simulink model "Posture_Regulation_Singularity_ROS"  (R2022b)
settings: Solver=FixedStepAuto  StartTime=0.0  StopTime=inf  FixedStep=0.02  MaxStep=0.1  RelTol=1e-3
undefined symbols (not defined in the file): theta_f, unicycle, X, x_f, Y, y_f
libraries: robotlib x3, simulink_extras x2
settings Model: Creator=Musta  LastModifiedBy=Musta
settings OptimizationCC: EnhancedBackFolding=on  PassReuseOutputArgsAs=Individual arguments  ZeroExternalMemoryAtStartup=off  ZeroInternalMemoryAtStartup=off  MaxStackSize=64  OptimizeBlockOrder=speed  DifferentSizesBufferReuse=on  OptimizationCustomize=off  EfficientTunableParamExpr=on
settings DebuggingCC: ParameterTunabilityLossMsg=error
settings HardwareCC: ProdBitPerPointer=32  ProdBitPerSizeT=32  ProdBitPerPtrDiffT=32  ProdLargestAtomicFloat=None  ProdIntDivRoundTo=Undefined  ProdEndianess=Unspecified  ProdWordSize=32  ProdHWDeviceType=Generic->Unspecified (assume 32-bit Generic)
settings SFSimCC: MATLABDynamicMemAlloc=off
settings RTWCC: Description=Embedded Coder  SystemTargetFile=ert.tlc  HardwareBoard=Robot Operating System (ROS)  TLCOptions="-aInlineSetEventsForThisBaseRateFcn=TLC_FALSE -aSuppressMultiTaskScheduler=TLC_FALSE  -aRateBasedStepFcn=0"  TemplateMakefile=ert_default_tmf  Toolchain=Catkin  TargetLang=C++
settings CodeAppCC: ForceParamTrailComments=on  IgnoreCustomStorageClasses=off  OperatorAnnotations=on  SimulinkDataObjDesc=on  SFDataObjDesc=on  InsertBlockDesc=on

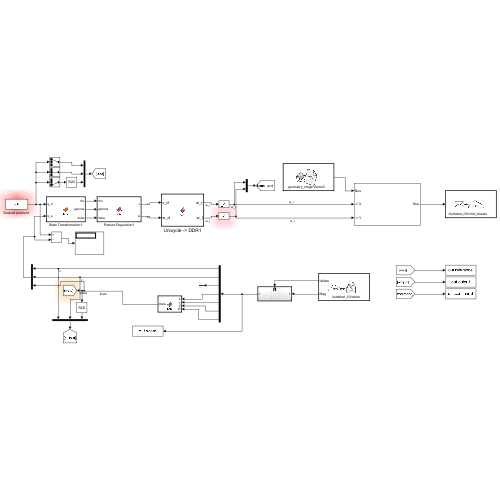
[thumbnail: Simulink's stored preview of the top-level diagram]
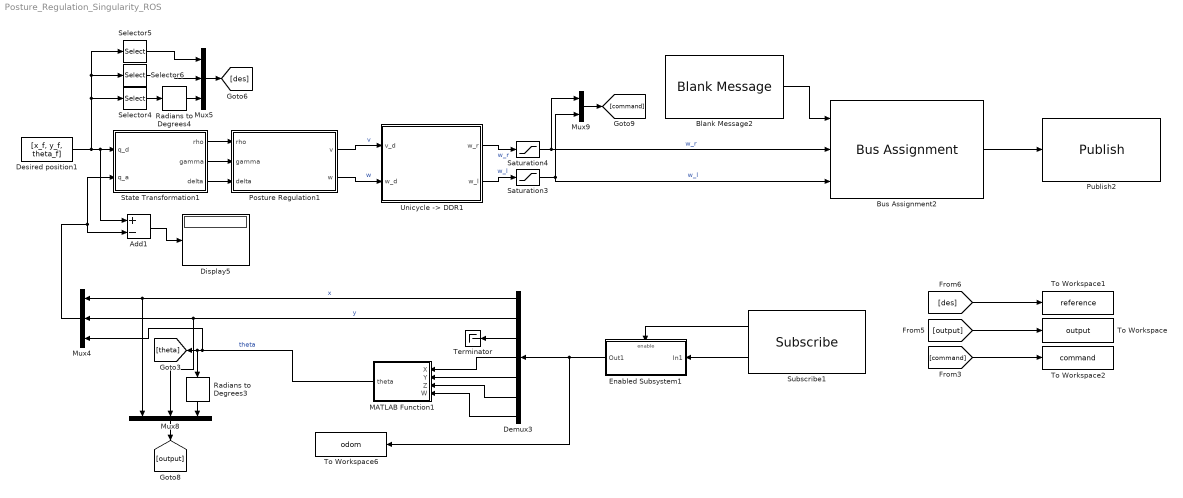
== system Posture_Regulation_Singularity_ROS ==
  Add1 : Sum  Inputs=+-
  Blank Message2 : robotlib/Blank Message  messageClass=Message  entityType=geometry_msgs/Vector3  messageType=geometry_msgs/Vector3  SampleTime=0.02  legacyBusStruct=off
      settings: LibrarySourceBlock=roslib/ROS/Blank Message
  Bus Assignment2 : BusAssignment  AssignedSignals=X,Y
  Demux3 : Demux  Outputs=7
  Desired position1 : Constant  Value=[x_f, y_f, theta_f]
  Display5 : Display
  Enabled Subsystem1 : Subsystem  TreatAsAtomicUnit=on
  MATLAB Function1 : MATLAB Function  TreatAsAtomicUnit=on
  Mux4 : Mux  Inputs=3
  Mux5 : Mux  Inputs=3
  Mux8 : Mux  Inputs=3
  Mux9 : Mux  Inputs=2
  Posture Regulation1 : MATLAB Function  TreatAsAtomicUnit=on
  Publish2 : robotlib/Publish  topicSource=Select from ROS network  topic=/turtlebot_03/cmd_wheels  messageType=geometry_msgs/Vector3  legacyBusStruct=off  messageQueueLength=1
      settings: LibrarySourceBlock=roslib/ROS/Publish
  Radians to Degrees3 : simulink_extras/Transformations/Radians to Degrees
  Radians to Degrees4 : simulink_extras/Transformations/Radians to Degrees
  Saturation3 : Saturate  UpperLimit=unicycle.omegaWheelMax  LowerLimit=unicycle.omegaWheelMin
  Saturation4 : Saturate  UpperLimit=13  LowerLimit=-13
  Selector4 : Selector  InputPortWidth=3  IndexOptions=Index vector (dialog)  Indices=3  OutputSizes=1
  Selector5 : Selector  InputPortWidth=3  IndexOptions=Index vector (dialog)  Indices=1  OutputSizes=1
  Selector6 : Selector  InputPortWidth=3  IndexOptions=Index vector (dialog)  Indices=2  OutputSizes=1
  State Transformation1 : MATLAB Function  TreatAsAtomicUnit=on
  Subscribe1 : robotlib/Subscribe  topicSource=Select from ROS network  topic=/turtlebot_03/odom  messageType=nav_msgs/Odometry  SampleTime=0.02  legacyBusStruct=off  messageQueueLength=1
      settings: LibrarySourceBlock=roslib/ROS/Subscribe
  Terminator : Terminator
  To Workspace : ToWorkspace  VariableName=output  SaveFormat=Structure With Time  SampleTime=-1
  To Workspace1 : ToWorkspace  VariableName=reference  SaveFormat=Structure With Time  SampleTime=-1
  To Workspace2 : ToWorkspace  VariableName=command  SaveFormat=Structure With Time  SampleTime=-1
  To Workspace6 : ToWorkspace  VariableName=odom  SaveFormat=Structure With Time  SampleTime=-1
  "Unicycle -> DDR1" : MATLAB Function  TreatAsAtomicUnit=on
  wires:
  [output] -> To Workspace/1
  [command] -> To Workspace2/1
  [des] -> To Workspace1/1
  Subscribe1/2 -> Enabled Subsystem1/1(In1)
  Enabled Subsystem1/1(Out1) -> Demux3/1, To Workspace6/1
  Subscribe1/1 -> Enabled Subsystem1/Enable
  MATLAB Function1/1(theta) -> Mux4/3, Radians to Degrees3/1, [theta]  "theta"
  Demux3/3 -> Terminator/1
  State Transformation1/1(rho) -> Posture Regulation1/1(rho)
  Demux3/1 -> Mux4/1, Mux8/1  "x"
  Selector5/1 -> Mux5/1
  Selector6/1 -> Mux5/2
  Radians to Degrees4/1 -> Mux5/3
  Mux5/1 -> [des]
  Bus Assignment2/1 -> Publish2/1
  Radians to Degrees3/1 -> Mux8/3
  Add1/1 -> Display5/1
  Demux3/2 -> Mux8/2, Mux4/2  "y"
  Posture Regulation1/1(v) -> "Unicycle -> DDR1"/1(v_d)  "v"
  Desired position1/1 -> Selector5/1, Selector6/1, Selector4/1, Add1/1, State Transformation1/1(q_d)
  Selector4/1 -> Radians to Degrees4/1
  State Transformation1/2(gamma) -> Posture Regulation1/2(gamma)
  Saturation4/1 -> Mux9/1, Bus Assignment2/2  "w_r"
  Mux4/1 -> State Transformation1/2(q_a), Add1/2
  Saturation3/1 -> Bus Assignment2/3, Mux9/2  "w_l"
  "Unicycle -> DDR1"/1(w_r) -> Saturation4/1  "w_r"
  Blank Message2/1 -> Bus Assignment2/1
  State Transformation1/3(delta) -> Posture Regulation1/3(delta)
  Posture Regulation1/2(w) -> "Unicycle -> DDR1"/2(w_d)  "w"
  Mux8/1 -> [output]
  "Unicycle -> DDR1"/2(w_l) -> Saturation3/1  "w_l"
  Mux9/1 -> [command]
  Demux3/5 -> MATLAB Function1/2(Y)
  Demux3/6 -> MATLAB Function1/3(Z)
  Demux3/4 -> MATLAB Function1/1(X)
  Demux3/7 -> MATLAB Function1/4(W)

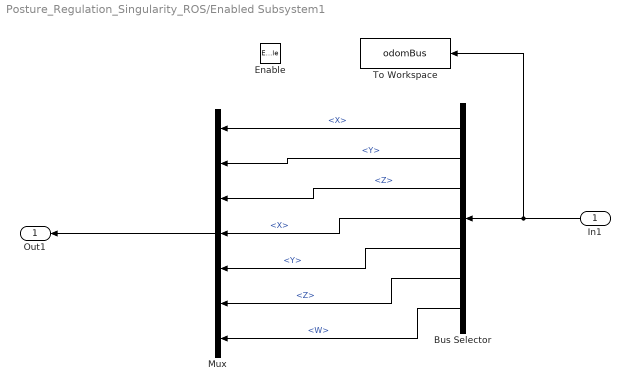
== system Posture_Regulation_Singularity_ROS/Enabled Subsystem1 ==
  In1 : Inport
  Enable : EnablePort
  Bus Selector : BusSelector  OutputSignals=Pose.Pose.Position.X,Pose.Pose.Position.Y,Pose.Pose.Position.Z,Pose.Pose.Orientation.X,Pose.Pose.Orientation.Y,Pose.Pose.Orientation.Z,Pose.Pose.Orientation.W
  Mux : Mux  Inputs=7
  To Workspace : ToWorkspace  VariableName=odomBus  SaveFormat=Timeseries  SampleTime=-1
  Out1 : Outport
  wires:
  Mux/1 -> Out1/1
  Bus Selector/1 -> Mux/1  "<X>"
  Bus Selector/2 -> Mux/2  "<Y>"
  In1/1 -> To Workspace/1, Bus Selector/1
  Bus Selector/3 -> Mux/3  "<Z>"
  Bus Selector/4 -> Mux/4  "<X>"
  Bus Selector/5 -> Mux/5  "<Y>"
  Bus Selector/6 -> Mux/6  "<Z>"
  Bus Selector/7 -> Mux/7  "<W>"

== matlab function Posture_Regulation_Singularity_ROS/MATLAB Function1 ==
  data: X input; theta output; Y input; Z input; W input
function theta = fcn(X, Y, Z, W)

    q_x = X;
    q_y = Y;
    q_z = Z;
    q_w = W;
    
    q = cat(2,q_x,q_y,q_z,q_w); 
    eulZYX = quat2eul(q,'ZYX');
    theta = eulZYX(:,3);
    
end

== matlab function Posture_Regulation_Singularity_ROS/Posture Regulation1 ==
  data: v output; w output; rho input; gamma input; delta input
function [v,w] = fcn(rho,gamma,delta)

    %#codegen
    coder.extrinsic('evalin')
    k1 = 0;                  % Needed in order to set variable class correctly
    k2 = 0;                  % Needed in order to set variable class correctly
    k3 = 0;                  % Needed in order to set variable class correctly
    k1 = evalin('base','k1'); % Read value from workspace
    k2 = evalin('base','k2'); % Read value from workspace
    k3 = evalin('base','k3'); % Read value from workspace

    v = k1 * rho * cos(gamma);
    w = k2 * gamma + k1 *(sin(gamma)*cos(gamma))*(gamma + k3 * delta)/gamma;

    % handling the singularity of v 
    if abs(v) < 10^-4
        if v > 0
            v = 10^-4;
        else
            v = -10^-4;
        end   
    end    

end

== matlab function Posture_Regulation_Singularity_ROS/State Transformation1 ==
  data: q_d input; rho output; q_a input; gamma output; delta output
function [rho,gamma,delta] = fcn(q_d, q_a)

    e_x = q_d(1) - q_a(1);
    e_y = q_d(2) - q_a(2);
    e_theta = q_d(3) - q_a(3);
   
    rho = sqrt(e_x^2 + e_y^2);
    gamma = mod(atan2(e_y,e_x),2*pi) - q_a(3);
    delta = gamma - e_theta;

%     e_x = q_d(1) - q_a(1);
%     e_y = q_d(2) - q_a(2);
%     e_theta = q_d(3) - q_a(3);
%    
%     rho = sqrt(e_x^2 + e_y^2);
% 
%     p = atan2(e_y,e_x);
%     % Count the number of turns around full circle
%     num_turns = floor(p/(2*pi));
%     % Adjust p to remove any full circle turns
%     theta_adj = p - num_turns*(2*pi);
% 
%     % gamma = mod(theta_adj,2*pi) - q_a(3);
%     gamma = theta_adj - q_a(3);
%     delta = gamma - e_theta;

end

== matlab function Posture_Regulation_Singularity_ROS/Unicycle -> DDR1 ==
  data: v_d input; w_r output; w_d input; w_l output
function [w_r, w_l] = fcn(v_d, w_d)

    %#codegen
    coder.extrinsic('evalin')
    d = 0;                  % Needed in order to set variable class correctly
    r = 0;                  % Needed in order to set variable class correctly
    d = evalin('base','unicycle.d'); % Read value from workspace
    r = evalin('base','unicycle.r'); % Read value from workspace

    w_r = ((2 * v_d) + (w_d * d)) / (2 * r);
    w_l = ((2 * v_d) - (w_d * d)) / (2 * r);

end
